simulink model "Simulink_Transformer_Model"  (R2021a)
settings: Solver=VariableStepAuto  StartTime=0.0  StopTime=0.2  RelTol=1e-3
libraries: spsLinearTransformerLib x4, spsGroundLib x2, spsBreakerLib x1, spsThreePhaseParallelRLCLoadLib x1, spsThreePhaseVIMeasurementLib x1, spsThreePhaseSourceLib x1, spspowerguiLib x1
settings Model: Creator=BIP  LastModifiedBy=BIP

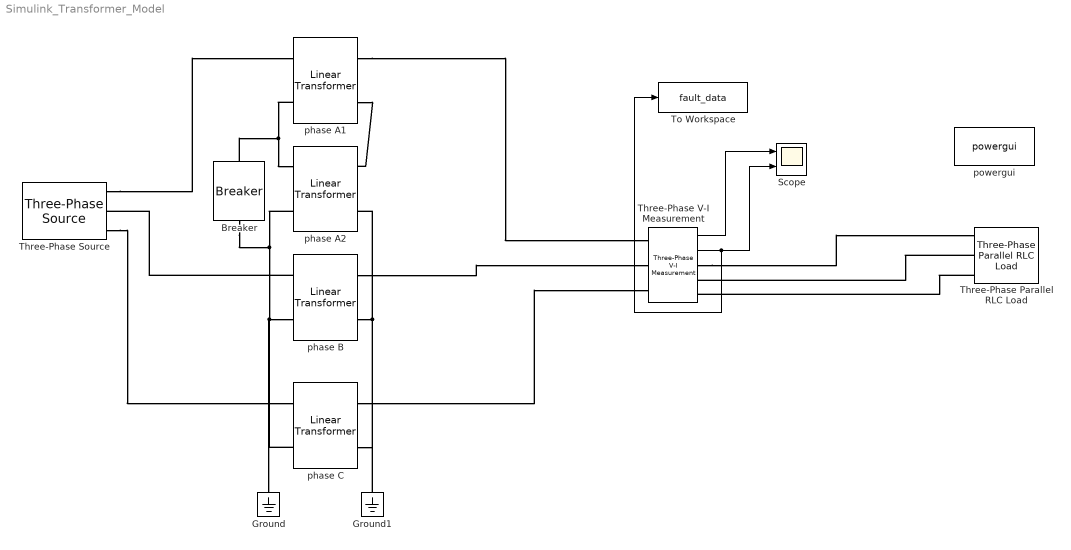
== system Simulink_Transformer_Model ==
  Breaker : spsBreakerLib/Breaker  InitialState=0  SwitchingTimes=T_fault  External=off  BreakerResistance=0.001  SnubberResistance=1e6  SnubberCapacitance=inf  Measurements=None  MoreParameters=on  NoBreakLoop=off
      settings: SourceProductBaseCode=PS
  Ground : spsGroundLib/Ground  LConnTagsString=a
  Ground1 : spsGroundLib/Ground  LConnTagsString=a
  Scope : Scope  NumInputPorts=2
  Three-Phase Parallel RLC Load : spsThreePhaseParallelRLCLoadLib/Three-Phase Parallel RLC Load  LConnTagsString=A|B|C  Configuration=Y (grounded)  NominalVoltage=400  Vabc=[1e3 1e3 1e3]  Vabcp=[1e3 1e3 1e3]  NominalFrequency=50  UnbalancedPower=off  ActivePower=10e6  InductivePower=1e6  CapacitivePower=0  Pabc=[10e3 9e3 11e3]  QLabc=[100 90 110]  QCabc=[100 90 110]  Pabcp=[10e3 9e3 11e3]  QLabcp=[100 90 110]  QCabcp=[100 90 110]  Measurements=None  LoadType=constant Z
  Three-Phase V-I Measurement : spsThreePhaseVIMeasurementLib/Three-Phase V-I Measurement  VoltageMeasurement=phase-to-ground  SetLabelV=off  LabelV=Vabc  Vpu=off  VpuLL=off  CurrentMeasurement=yes  SetLabelI=off  LabelI=Iabc  Ipu=off  Pbase=100e6  Vbase=500e3  OutputType=Complex  PhasorSimulation=off  PSBequivalent=0
  Three-Phase Source : spsThreePhaseSourceLib/Three-Phase Source  InternalConnection=Yg  VoltagePhases=off  Voltage=20e3  PhaseAngle=0  Voltage_phases=[25e3 25e3 25e3]/sqrt(3)  PhaseAngles_phases=[0 -120 +120]  Frequency=50  NonIdealSource=on  SpecifyImpedance=off  Resistance=0.8929  Inductance=16.58e-3  ShortCircuitLevel=100e6  BaseVoltage=20e3  XRratio=7  BusType=swing  Pref=10e3  Qref=0  Prefabc=[10e3, 10e3, 10e3]  Qrefabc=[0, 0, 0]  Qmin=-inf  Qmax=inf
  To Workspace : ToWorkspace  VariableName=fault_data  SaveFormat=Structure With Time  SampleTime=-1
  phase A1 : spsLinearTransformerLib/Linear Transformer  UNITS=pu  NominalPower=[ 31.66e6 50 ]  winding1="[ 0.95 * (20000/sqrt(3))  0.002  0.08 ]"  winding2="[ 0.95 * (400/sqrt(3))  0.002  0.08 ]"  ThreeWindings=off  winding3=[ 0 0 0 ]  RmLm=[ 500 500 ]  Measurements=None  DataType=off
  phase A2 : spsLinearTransformerLib/Linear Transformer  UNITS=pu  NominalPower=[ 1.66e6 50 ]  winding1="[ 0.05 * (20000/sqrt(3))  0.002  0.08 ]"  winding2="[ 0.05 * (400/sqrt(3))  0.002  0.08 ]"  ThreeWindings=off  winding3=[ 0 0 0 ]  RmLm=[ 500 500 ]  Measurements=None  DataType=off
  phase B : spsLinearTransformerLib/Linear Transformer  UNITS=pu  NominalPower=[ 33.33e6 50 ]  winding1=[20000/sqrt(3) , 0.002 , 0.08]  winding2=[400/sqrt(3) , 0.002 , 0.08]  ThreeWindings=off  winding3=[ 0 0 0 ]  RmLm=[500 500]  Measurements=None  DataType=off
  phase C : spsLinearTransformerLib/Linear Transformer  UNITS=pu  NominalPower=[ 33.33e6 50 ]  winding1=[20000/sqrt(3) , 0.002 , 0.08]  winding2=[400/sqrt(3) , 0.002 , 0.08]  ThreeWindings=off  winding3=[ 0 0 0 ]  RmLm=[ 500 500 ]  Measurements=None  DataType=off
  powergui : spspowerguiLib/powergui  Priority=1  SimulationMode=Continuous  SampleTime=50e-6  frequency=60  Iterations=50  frequencyindice=50  Pbase=100e6  ErrMax=1e-4  UnitsV=kV  UnitsW=MW  buscounter=0  FunctionMessages=off  echomessages=off  EnableUseOfTLC=off  CurrentSourceSwitches=off  DisableSnubberDevices=off  DisableRonSwitches=off  DisableVfSwitches=off  DisplayEquations=off  AutomaticDiscreteSolvers=off  SolverType=Tustin/Backward Euler (TBE)  Interpol=off  ExternalGateDelay=off  methode=off  Ts=100  x0status=blocks  SPID=on  SwTol=0  HookPort=off  NonlinearTolerance=1e-4  nMaxIteration=100  ContinueOnMaxIteration=off  RestoreLinks=warning  ResistiveCurrentMeasurement=off  Frange=[0:2:500]  Ylog=off  Xlog=on  ShowGrid=off  save=off  variable=ZData  structure=0  ZoomFFT=off  StartTime=0.0  cycles=1  DisplayStyle=1  fundamental=60  FreqAxis=off  MaxFrequency=1000  frequencyindicesteady=1  RmsSteady=1  display=off
  wires:
  Three-Phase V-I Measurement/1 -> Scope/1
  Three-Phase V-I Measurement/2 -> Scope/2, To Workspace/1
  connections:
  phase A1/LConn2 -- phase A2/LConn1 -- Breaker/LConn1
  Three-Phase Source/RConn1 -- phase A1/LConn1
  phase B/LConn1 -- Three-Phase Source/RConn2
  Three-Phase Source/RConn3 -- phase C/LConn1
  phase A2/LConn2 -- Breaker/RConn1 -- Ground/LConn1 -- phase C/LConn2 -- phase B/LConn2
  phase A1/RConn2 -- phase A2/RConn1
  phase B/RConn2 -- Ground1/LConn1 -- phase C/RConn2 -- phase A2/RConn2
  Three-Phase V-I Measurement/RConn1 -- Three-Phase Parallel RLC Load/LConn1
  Three-Phase Parallel RLC Load/LConn2 -- Three-Phase V-I Measurement/RConn2
  Three-Phase Parallel RLC Load/LConn3 -- Three-Phase V-I Measurement/RConn3
  phase A1/RConn1 -- Three-Phase V-I Measurement/LConn1
  phase B/RConn1 -- Three-Phase V-I Measurement/LConn2
  phase C/RConn1 -- Three-Phase V-I Measurement/LConn3
